simulink model "main_eps"  (R2021b)
settings: Solver=FixedStepDiscrete  StartTime=0.0  StopTime=10.0  FixedStep=0.1  RelTol=1e-3  EnableMultiTasking=on
settings Model: Creator=User  LastModifiedBy=User
settings SolverCC: AlgebraicLoopSolver=TrustRegion  AutoInsertRateTranBlk=on
settings DataIOCC: LimitDataPoints=on
settings OptimizationCC: LifeSpan=inf
settings DebuggingCC: AllowSymbolicDim=off  SFUnexpectedBacktrackingDiag=warning  SFNoUnconditionalDefaultTransitionDiag=warning  SFExecutionAtInitializationDiag=none  ArithmeticOperatorsInVariantConditions=warning
settings SFSimCC: SimUseLocalCustomCode=off  CustomCodeUndefinedFunction=UseInterfaceOnly
settings RTWCC: RTWUseLocalCustomCode=off
settings CodeAppCC: StateflowObjectComments=on
settings GRTTargetCC: TargetLangStandard=C89/C90 (ANSI)
settings ConfigComp: CovMetricSettings=dw  CovSaveCumulativeToWorkspaceVar=on  CovSaveSingleToWorkspaceVar=on  CovExternalEMLEnable=off  CovSFcnEnable=off

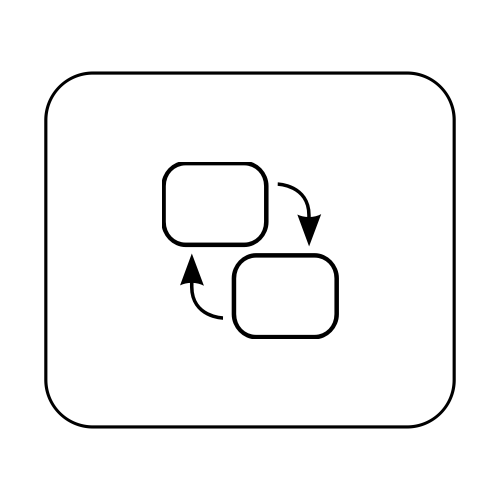
[thumbnail: Simulink's stored preview of the top-level diagram]
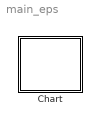
== system main_eps ==
  Chart : Stateflow chart  TreatAsAtomicUnit=on

== stateflow chart main_eps/Chart ==
  state Bateria_PS
  state Seguranca
  state Normal_Sol
  state Normal_Eclipse
  state Bateria_Cheia
  (junction 33) -> (junction 32) : %[Iluminado == 1]
  (junction 32) -> Bateria_PS
  (junction 30) -> (junction 33) [order 1]
  Bateria_PS -> (junction 21) [order 1] : %[Iluminado == 0]
  Bateria_PS -> (junction 42) [order 3] : %[TC_SAFE == 1]
      | %TC_SSAFE é acionado com alguma
      | %condição de Cbat
  (junction 21) -> Normal_Eclipse
  (junction 42) -> Seguranca
  Normal_Sol -> Bateria_PS [order 2] : %[Ppainel < Pcargas]
  Bateria_PS -> Normal_Sol [order 2] : %[Ppainel > Pcargas]
  (default) -> Seguranca
  Seguranca -> Normal_Sol : %[Iluminado == 1 && Cbat <100 && Ppainel > Pcargas]
  Normal_Sol -> Normal_Eclipse [order 3] : %[Iluminado == 0]
  Normal_Eclipse -> (junction 30)
  (junction 30) -> (junction 45) [order 2]
  (junction 46) -> Seguranca
  Normal_Sol -> Bateria_Cheia [order 1] : %[Cbat == 100]
  Bateria_Cheia -> Normal_Sol [order 2] : %[Cbat <100]
  (junction 22) -> Normal_Eclipse
  Bateria_Cheia -> (junction 22) [order 1] : %[Iluminado == 0]
  (junction 45) -> (junction 46) : %[TC_SAFE == 1]
      | %TC_SSAFE é acionado com alguma
      | %condição de Cbat
